simulink model "Punto1a_triangular_0_1rad"  (Simulink 7.5)
settings: Solver=ode45  StartTime=0  StopTime=140  MaxStep=1  RelTol=1e-3
libraries: simulink x1
settings Model: Creator=Nahuek  LastModifiedBy=Nahuek

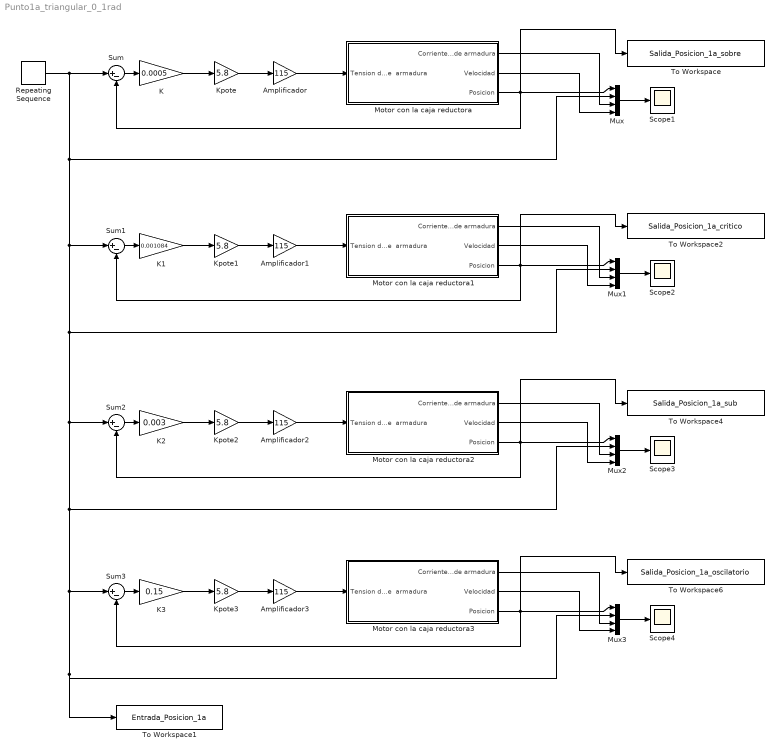
== system Punto1a_triangular_0_1rad ==
  Amplificador{,1..3} (4 alike) : Gain  Gain=115  ParameterDataType=fixdt(1, 16)  ParameterScaling=2^0  OutDataType=fixdt(1, 16)  OutScaling=2^0
  K : Gain  Gain=0.0005  ParameterDataType=fixdt(1, 16)  ParameterScaling=2^0  OutDataType=fixdt(1, 16)  OutScaling=2^0
  K1 : Gain  Gain=0.001084  ParameterDataType=fixdt(1, 16)  ParameterScaling=2^0  OutDataType=fixdt(1, 16)  OutScaling=2^0
  K2 : Gain  Gain=0.003  ParameterDataType=fixdt(1, 16)  ParameterScaling=2^0  OutDataType=fixdt(1, 16)  OutScaling=2^0
  K3 : Gain  Gain=0.15  ParameterDataType=fixdt(1, 16)  ParameterScaling=2^0  OutDataType=fixdt(1, 16)  OutScaling=2^0
  Kpote{,1..3} (4 alike) : Gain  Gain=5.8  ParameterDataType=fixdt(1, 16)  ParameterScaling=2^0  OutDataType=fixdt(1, 16)  OutScaling=2^0
  Motor con la caja reductora : Subsystem
  Motor con la caja reductora1 : Subsystem
  Motor con la caja reductora2 : Subsystem
  Motor con la caja reductora3 : Subsystem
  Mux{,1..3} (4 alike) : Mux
  Repeating Sequence : simulink/Sources/Repeating Sequence  SystemSampleTime=-1  rep_seq_t=[0 31.4159 62.8319]  rep_seq_y=[-1 1 -1]
  Scope{1..4} (4 alike) : Scope
      Scope1 settings: TickLabels=on  TimeRange=200  YMin=0  YMax=1.4
      Scope2 settings: TickLabels=on  TimeRange=200  YMin=0  YMax=1.1
      Scope3 settings: TickLabels=on  TimeRange=10  YMin=0  YMax=1.1  SaveName=ScopeData2
      Scope4 settings: TickLabels=on  TimeRange=10  YMin=0  YMax=1.1  SaveName=ScopeData3
  Sum{,1..3} (4 alike) : Sum  Inputs=|+-  OutDataType=fixdt(1, 16)  OutScaling=2^0
  To Workspace : ToWorkspace  VariableName=Salida_Posicion_1a_sobre  SampleTime=-1  SaveFormat=Structure With Time
  To Workspace1 : ToWorkspace  VariableName=Entrada_Posicion_1a  SampleTime=-1  SaveFormat=Structure With Time
  To Workspace2 : ToWorkspace  VariableName=Salida_Posicion_1a_critico  SampleTime=-1  SaveFormat=Structure With Time
  To Workspace4 : ToWorkspace  VariableName=Salida_Posicion_1a_sub  SampleTime=-1  SaveFormat=Structure With Time
  To Workspace6 : ToWorkspace  VariableName=Salida_Posicion_1a_oscilatorio  SampleTime=-1  SaveFormat=Structure With Time
  wires:
  Mux/1 -> Scope1/1
  Repeating Sequence/1 -> Sum/1, Sum1/1, Sum2/1, Sum3/1, Mux3/2, To Workspace1/1, Mux2/2, Mux1/2, Mux/2
  Sum/1 -> K/1
  K/1 -> Kpote/1
  Kpote/1 -> Amplificador/1
  Amplificador/1 -> Motor con la caja reductora/1(Tension de  armadura)
  Motor con la caja reductora/3(Posicion) -> Mux/1, Sum/2, To Workspace/1
  Mux1/1 -> Scope2/1
  Sum1/1 -> K1/1
  K1/1 -> Kpote1/1
  Kpote1/1 -> Amplificador1/1
  Amplificador1/1 -> Motor con la caja reductora1/1(Tension de  armadura)
  Motor con la caja reductora1/3(Posicion) -> Mux1/1, Sum1/2, To Workspace2/1
  Mux2/1 -> Scope3/1
  Sum2/1 -> K2/1
  K2/1 -> Kpote2/1
  Kpote2/1 -> Amplificador2/1
  Amplificador2/1 -> Motor con la caja reductora2/1(Tension de  armadura)
  Motor con la caja reductora2/3(Posicion) -> Mux2/1, Sum2/2, To Workspace4/1
  Mux3/1 -> Scope4/1
  Sum3/1 -> K3/1
  K3/1 -> Kpote3/1
  Kpote3/1 -> Amplificador3/1
  Amplificador3/1 -> Motor con la caja reductora3/1(Tension de  armadura)
  Motor con la caja reductora3/3(Posicion) -> Mux3/1, Sum3/2, To Workspace6/1
  Motor con la caja reductora3/1(Corriente de armadura) -> Mux3/3
  Motor con la caja reductora3/2(Velocidad) -> Mux3/4
  Motor con la caja reductora2/1(Corriente de armadura) -> Mux2/3
  Motor con la caja reductora2/2(Velocidad) -> Mux2/4
  Motor con la caja reductora1/1(Corriente de armadura) -> Mux1/3
  Motor con la caja reductora1/2(Velocidad) -> Mux1/4
  Motor con la caja reductora/1(Corriente de armadura) -> Mux/3
  Motor con la caja reductora/2(Velocidad) -> Mux/4

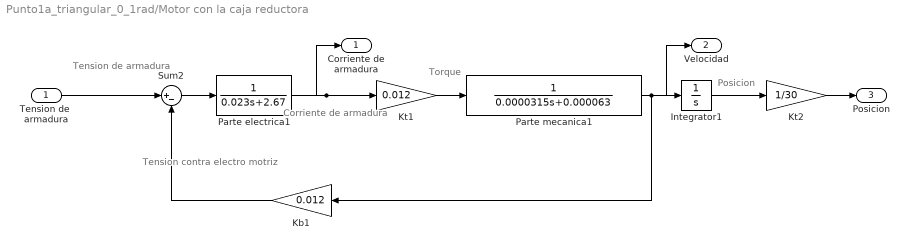
== system Punto1a_triangular_0_1rad/Motor con la caja reductora ==
  note: Tension contra
      |  electro motriz
  note: Corriente de
      | armadura
  note: Torque
  note: Posicion
  note: Tension de
      |  armadura
  Tension de  armadura : Inport
  Integrator1 : Integrator
  Kb1 : Gain  Gain=0.012  ParameterDataType=fixdt(1, 16)  ParameterScaling=2^0  OutDataType=fixdt(1, 16)  OutScaling=2^0
  Kt1 : Gain  Gain=0.012  ParameterDataType=fixdt(1, 16)  ParameterScaling=2^0  OutDataType=fixdt(1, 16)  OutScaling=2^0
  Kt2 : Gain  Gain=1/30  ParameterDataType=fixdt(1, 16)  ParameterScaling=2^0  OutDataType=fixdt(1, 16)  OutScaling=2^0
  Parte electrica1 : TransferFcn  Denominator=[0.023 2.67]
  Parte mecanica1 : TransferFcn  Denominator=[0.0000315 0.000063]
  Sum2 : Sum  Inputs=|+-  OutDataType=fixdt(1, 16)  OutScaling=2^0
  Corriente de armadura : Outport
  Velocidad : Outport  Port=2
  Posicion : Outport  Port=3
  wires:
  Sum2/1 -> Parte electrica1/1
  Kt1/1 -> Parte mecanica1/1
  Parte electrica1/1 -> Kt1/1, Corriente de armadura/1
  Kb1/1 -> Sum2/2
  Parte mecanica1/1 -> Integrator1/1, Kb1/1, Velocidad/1
  Tension de  armadura/1 -> Sum2/1
  Kt2/1 -> Posicion/1
  Integrator1/1 -> Kt2/1

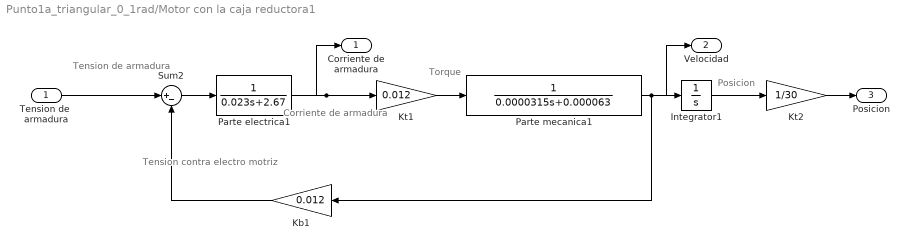
== system Punto1a_triangular_0_1rad/Motor con la caja reductora1 ==
  note: Tension contra
      |  electro motriz
  note: Corriente de
      | armadura
  note: Torque
  note: Posicion
  note: Tension de
      |  armadura
  Tension de  armadura : Inport
  Integrator1 : Integrator
  Kb1 : Gain  Gain=0.012  ParameterDataType=fixdt(1, 16)  ParameterScaling=2^0  OutDataType=fixdt(1, 16)  OutScaling=2^0
  Kt1 : Gain  Gain=0.012  ParameterDataType=fixdt(1, 16)  ParameterScaling=2^0  OutDataType=fixdt(1, 16)  OutScaling=2^0
  Kt2 : Gain  Gain=1/30  ParameterDataType=fixdt(1, 16)  ParameterScaling=2^0  OutDataType=fixdt(1, 16)  OutScaling=2^0
  Parte electrica1 : TransferFcn  Denominator=[0.023 2.67]
  Parte mecanica1 : TransferFcn  Denominator=[0.0000315 0.000063]
  Sum2 : Sum  Inputs=|+-  OutDataType=fixdt(1, 16)  OutScaling=2^0
  Corriente de armadura : Outport
  Velocidad : Outport  Port=2
  Posicion : Outport  Port=3
  wires:
  Sum2/1 -> Parte electrica1/1
  Kt1/1 -> Parte mecanica1/1
  Parte electrica1/1 -> Kt1/1, Corriente de armadura/1
  Kb1/1 -> Sum2/2
  Parte mecanica1/1 -> Integrator1/1, Kb1/1, Velocidad/1
  Tension de  armadura/1 -> Sum2/1
  Kt2/1 -> Posicion/1
  Integrator1/1 -> Kt2/1

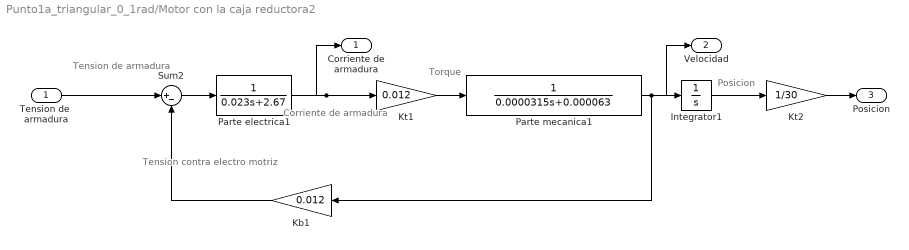
== system Punto1a_triangular_0_1rad/Motor con la caja reductora2 ==
  note: Tension contra
      |  electro motriz
  note: Corriente de
      | armadura
  note: Torque
  note: Posicion
  note: Tension de
      |  armadura
  Tension de  armadura : Inport
  Integrator1 : Integrator
  Kb1 : Gain  Gain=0.012  ParameterDataType=fixdt(1, 16)  ParameterScaling=2^0  OutDataType=fixdt(1, 16)  OutScaling=2^0
  Kt1 : Gain  Gain=0.012  ParameterDataType=fixdt(1, 16)  ParameterScaling=2^0  OutDataType=fixdt(1, 16)  OutScaling=2^0
  Kt2 : Gain  Gain=1/30  ParameterDataType=fixdt(1, 16)  ParameterScaling=2^0  OutDataType=fixdt(1, 16)  OutScaling=2^0
  Parte electrica1 : TransferFcn  Denominator=[0.023 2.67]
  Parte mecanica1 : TransferFcn  Denominator=[0.0000315 0.000063]
  Sum2 : Sum  Inputs=|+-  OutDataType=fixdt(1, 16)  OutScaling=2^0
  Corriente de armadura : Outport
  Velocidad : Outport  Port=2
  Posicion : Outport  Port=3
  wires:
  Sum2/1 -> Parte electrica1/1
  Kt1/1 -> Parte mecanica1/1
  Parte electrica1/1 -> Kt1/1, Corriente de armadura/1
  Kb1/1 -> Sum2/2
  Parte mecanica1/1 -> Integrator1/1, Kb1/1, Velocidad/1
  Tension de  armadura/1 -> Sum2/1
  Kt2/1 -> Posicion/1
  Integrator1/1 -> Kt2/1

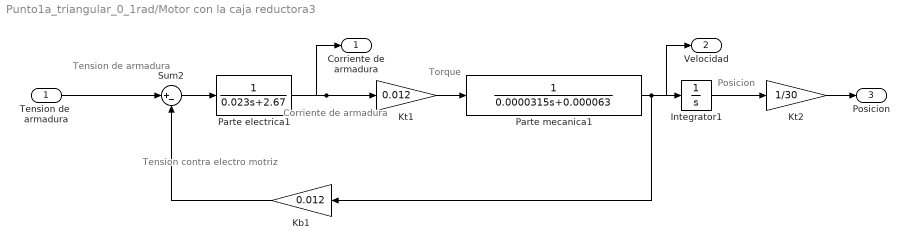
== system Punto1a_triangular_0_1rad/Motor con la caja reductora3 ==
  note: Tension contra
      |  electro motriz
  note: Corriente de
      | armadura
  note: Torque
  note: Posicion
  note: Tension de
      |  armadura
  Tension de  armadura : Inport
  Integrator1 : Integrator
  Kb1 : Gain  Gain=0.012  ParameterDataType=fixdt(1, 16)  ParameterScaling=2^0  OutDataType=fixdt(1, 16)  OutScaling=2^0
  Kt1 : Gain  Gain=0.012  ParameterDataType=fixdt(1, 16)  ParameterScaling=2^0  OutDataType=fixdt(1, 16)  OutScaling=2^0
  Kt2 : Gain  Gain=1/30  ParameterDataType=fixdt(1, 16)  ParameterScaling=2^0  OutDataType=fixdt(1, 16)  OutScaling=2^0
  Parte electrica1 : TransferFcn  Denominator=[0.023 2.67]
  Parte mecanica1 : TransferFcn  Denominator=[0.0000315 0.000063]
  Sum2 : Sum  Inputs=|+-  OutDataType=fixdt(1, 16)  OutScaling=2^0
  Corriente de armadura : Outport
  Velocidad : Outport  Port=2
  Posicion : Outport  Port=3
  wires:
  Sum2/1 -> Parte electrica1/1
  Kt1/1 -> Parte mecanica1/1
  Parte electrica1/1 -> Kt1/1, Corriente de armadura/1
  Kb1/1 -> Sum2/2
  Parte mecanica1/1 -> Integrator1/1, Kb1/1, Velocidad/1
  Tension de  armadura/1 -> Sum2/1
  Kt2/1 -> Posicion/1
  Integrator1/1 -> Kt2/1
